simulink model "timer1"  (Simulink 8.0)
settings: Solver=ode45  StartTime=0.0  StopTime=inf  RelTol=1e-3
libraries: dspswit3 x2, simulink x1
settings Model: Creator=Eka  LastModifiedBy=Wk
settings DataIOCC: SignalLoggingSaveFormat=ModelDataLogs
settings DebuggingCC: FcnCallInpInsideContextMsg=UseLocalSettings
settings GRTTargetCC: CombineOutputUpdateFcns=off  GRTInterface=on
settings ConfigurationSet: Description=SimMechanics 2G
settings SimEventsCC: propDiagAttribOutput=1  propDiagFcnCallOutput=1  propDiagStatOutput=0  propPreventDuplicateEvents=0

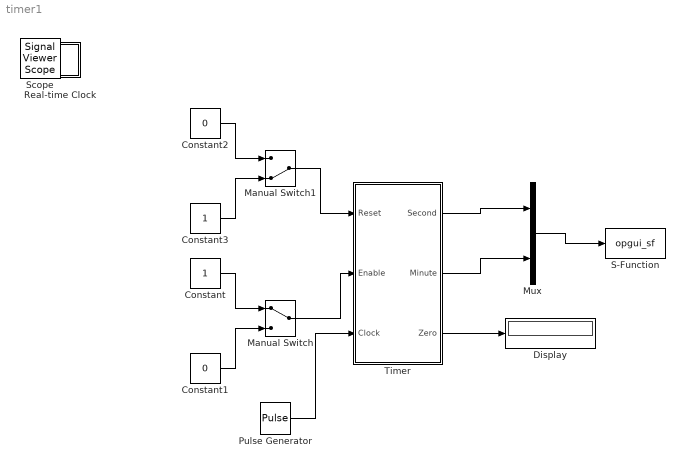
== system timer1 ==
  Constant : Constant
  Constant1 : Constant  Value=0
  Constant2 : Constant  Value=0
  Constant3 : Constant
  Display : Display
  Manual Switch : ManualSwitch
  Manual Switch1 : ManualSwitch  CurrentSetting=0
  Mux : Mux  Inputs=2
  Pulse Generator : DiscretePulseGenerator  PulseType=Time based  Period=1  PulseWidth=50
  Real-time Clock : Subsystem  mask(Real-time Clock){sample_time=0.02, tolerance=1}
      mask prompts: sample_time "Synchronize with real-time every n seconds:"; tolerance "Real-time warning tolerance (seconds):"
      mask help: Real-time Synchronization Block
      mask Help: This block synchronizes simulation time with the PC real-time clock or UNIX system clock. The first dialog entry is the period at which the clock is checked to insure real-time synchronization. The second dialog entry is the number of seconds that the simulation time must be within real-time before a warning is printed.
      mask Display: plot(0,0,100,100,[40,60,60,54,54,64,69,76,82,77,81,83,83,81,78,74,70,64,57,49,41,35,32,30,30,31,34,40,47,47,40,40],[90,90,85,85,80,79,76,87,80,70,64,57,49,41,33,28,24,22,21,23,25,31,37,46,56,65,73,78,80,85,85,90],[69,53,53],[64,50,73])
  S-Function : S-Function  FunctionName=opgui_sf  Parameters=0.005  EnableBusSupport=off
  Timer : Subsystem
  Scope : SignalViewerScope  IOType=viewer  RefreshTime=0.035000
      settings: YMin=0  YMax=60
  wires:
  Constant/1 -> Manual Switch/1
  Constant1/1 -> Manual Switch/2
  Manual Switch/1 -> Timer/2(Enable)
  Constant2/1 -> Manual Switch1/1
  Constant3/1 -> Manual Switch1/2
  Manual Switch1/1 -> Timer/1(Reset)
  Pulse Generator/1 -> Timer/3(Clock)
  Timer/1(Second) -> Mux/1
  Timer/2(Minute) -> Mux/2
  Mux/1 -> S-Function/1
  Timer/3(Zero) -> Display/1

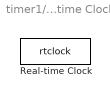
== system timer1/Real-time Clock ==
  Real-time Clock : S-Function  FunctionName=rtclock  Parameters=sample_time, tolerance  EnableBusSupport=off

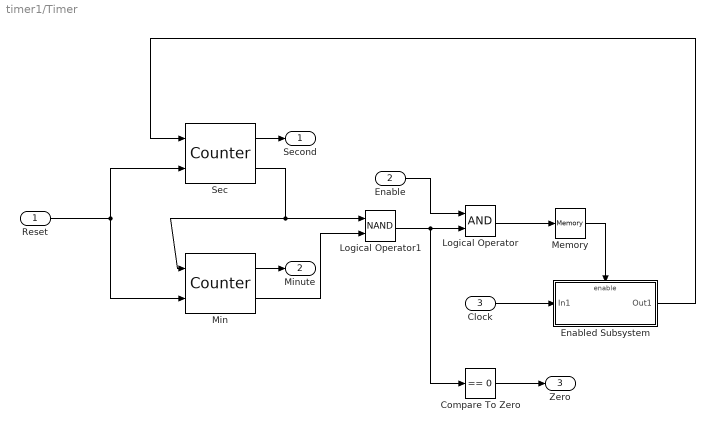
== system timer1/Timer ==
  Reset : Inport
  Enable : Inport  Port=2
  Clock : Inport  Port=3
  Compare To Zero : simulink/Logic and Bit Operations/Compare To Zero  relop===  OutDataTypeStr=uint8
  Enabled Subsystem : Subsystem  TreatAsAtomicUnit=on
  Logical Operator : Logic  AllPortsSameDT=off  OutDataTypeStr=boolean
  Logical Operator1 : Logic  Operator=NAND  AllPortsSameDT=off  OutDataTypeStr=boolean
  Memory : Memory
  Min : dspswit3/Counter  Direction=Down  CountEvent=Falling edge  CounterSize=User defined  MaxCount=255  InitialCount=0  Output=Count and Hit  HitValue=0  ResetInput=on  SamplesPerFrame=1  Ts=1  CntDtype=double  HitDtype=Logical
  Sec : dspswit3/Counter  Direction=Down  CountEvent=Falling edge  CounterSize=User defined  MaxCount=59  InitialCount=6  Output=Count and Hit  HitValue=0  ResetInput=on  SamplesPerFrame=1  Ts=1  CntDtype=double  HitDtype=Logical
  Second : Outport
  Minute : Outport  Port=2
  Zero : Outport  Port=3
  wires:
  Sec/2 -> Min/1, Logical Operator1/1
  Min/2 -> Logical Operator1/2
  Reset/1 -> Sec/2, Min/2
  Memory/1 -> Enabled Subsystem/Enable
  Enable/1 -> Logical Operator/1
  Logical Operator1/1 -> Logical Operator/2, Compare To Zero/1
  Logical Operator/1 -> Memory/1
  Enabled Subsystem/1(Out1) -> Sec/1
  Min/1 -> Minute/1
  Sec/1 -> Second/1
  Compare To Zero/1 -> Zero/1
  Clock/1 -> Enabled Subsystem/1(In1)

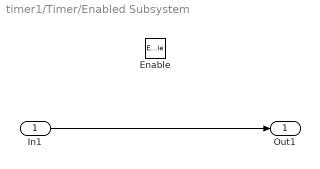
== system timer1/Timer/Enabled Subsystem ==
  In1 : Inport
  Enable : EnablePort
  Out1 : Outport
  wires:
  In1/1 -> Out1/1
